simulink model "flexcan_can_fd_master_s32k14_Main_1"  (R2017a)
settings: Solver=FixedStepDiscrete  StartTime=0.0  StopTime=10.0  FixedStep=0.1  RelTol=1e-3  EnableMultiTasking=on
InitFcn:
  | mbd_s32k14_consistency_checks(bdroot(gcs));
undefined symbols (not defined in the file): A9, AD0, B8, C10, C2, C7, D1, D2, H6, PTA0, PTA2, PTC15, PTC6, PTC7, PTD0, PTE4, PTE5
libraries: mbd_s32k14_ec_toolbox x9
Description:
  | This model tests FlexCAN communication using CAN with Flexible Data-Rate.
  | The FlexCAN Master sends on each step a message with ID 0x3FF to the slave.
  | On each Tx Complete event Blue LED (PTD0) is toggled.
  | 
  | HW prerequisite:
  | - S32K144EVB-Q100
  | - Make sure that J107 has pin 1 and 2 connected and external power supply is provieded through J16.
  | 
  | Validation:
  | - The CAN Baudrate is set to 500 Kb/s
  | - Any CAN analizer (USB to CAN device) can be used to observe CAN traffic via board CAN port J13.
settings Model: Creator=agrigorev  LastModifiedBy=sreer
settings DataIOCC: ExternalInput=off  InitialState=off  LimitDataPoints=on  SaveFormat=Array  SaveOutput=off  SignalLogging=off  SaveTime=off
settings OptimizationCC: DefaultParameterBehavior=Inlined  PassReuseOutputArgsAs=Individual arguments
settings DebuggingCC: UnderspecifiedInitializationDetection=Classic  MergeDetectMultiDrivingBlocksExec=none  SolverPrmCheckMsg=warning  InheritedTsInSrcMsg=none  SingleTaskRateTransMsg=error  ParameterTunabilityLossMsg=error  UnconnectedInputMsg=error  UnconnectedOutputMsg=error  UnconnectedLineMsg=error  AllowSymbolicDim=off  UnknownTsInhSupMsg=error  StateNameClashWarn=warning  SFUnexpectedBacktrackingDiag=warning  SFNoUnconditionalDefaultTransitionDiag=warning  SFExecutionAtInitializationDiag=none
settings HardwareCC: ProdBitPerPointer=32  ProdBitPerSizeT=32  ProdBitPerPtrDiffT=32  ProdLargestAtomicInteger=Long  ProdLargestAtomicFloat=Double  ProdWordSize=32  ProdHWDeviceType=ARM Compatible->ARM Cortex
settings ModelReferenceCC: PropagateSignalLabelsOutOfModel=off
settings SFSimCC: MATLABDynamicMemAlloc=off
settings RTWCC: SystemTargetFile=mbd_s32k14.tlc  MakeCommand=mbd_s32k14_make_rtw COPY_MDLREF_INCLUDES=0  TemplateMakefile=mbd_s32k14.tmf  Description=Model Based Design Toolbox S32K14x Code Generation Target  GenerateReport=on  IncludeHyperlinkInReport=on  LaunchReport=on  GenerateTraceInfo=on  GenerateTraceReport=on  GenerateTraceReportSl=on  GenerateTraceReportSf=on  GenerateTraceReportEml=on
settings CodeAppCC: ForceParamTrailComments=on  IgnoreCustomStorageClasses=off  OperatorAnnotations=on  SimulinkDataObjDesc=on  SFDataObjDesc=on  MATLABFcnDesc=on  InsertBlockDesc=on  MATLABSourceComments=on
settings STFCustomTargetCC: MultiwordLength=256  CombineOutputUpdateFcns=on  ERTCustomFileBanners=on  SupportContinuousTime=off  SupportNonInlinedSFcns=off  RemoveResetFunc=on  MATLABClassNameForMDSCustomization=Simulink.SoftwareTarget.ERTCustomization  GRTInterface=off  SystemTargetFile=mbd_s32k14.tlc
settings ERTTargetCC: ParMdlRefBuildCompliant=off  CompOptLevelCompliant=off  ConcurrentExecutionCompliant=off  ERTFirstTimeCompliant=off  ModelStepFunctionPrototypeControlCompliant=off  CPPClassGenCompliant=off  UseToolchainInfoCompliant=off  InlinedParameterPlacement=NonHierarchical  ERTCustomFileTemplate=example_file_process.tlc
settings ConfigComp: CovMetricSettings=dw  CovHtmlReporting=on  CovSaveCumulativeToWorkspaceVar=on  CovSaveSingleToWorkspaceVar=on  CovExternalEMLEnable=off

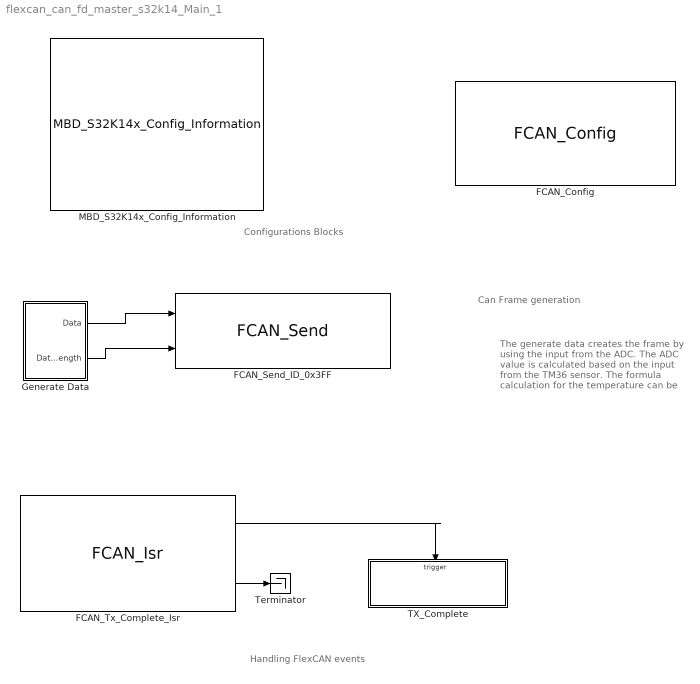
== system flexcan_can_fd_master_s32k14_Main_1 ==
  note: Handling FlexCAN events
  note: The generate data creates the frame by using the input from the ADC. The ADC value is calculated based on the input from the TM36 sensor. The formula calculation for the temperature can be
  note: Can Frame generation
  note: Configurations Blocks
  FCAN_Config : mbd_s32k14_ec_toolbox/S32K14x/Communication Blocks/Flex CAN Blocks/FCAN_Config  Priority=1  can_instance=0  can_mode=Normal mode  can_max_num_mb=16  can_rx=PTE4 : [9] : [6] : [D1]  can_tx=PTE5 : [8] : [5] : [D2]  show_adv_opts=on  can_clk_src=Peripheral clock  can_presdiv=9  can_rjw=0  can_pseg1=3  can_pseg2=3  can_propseg=6  can_cbt_presdiv=9  can_cbt_rjw=0  can_cbt_pseg1=3  can_cbt_pseg2=3  can_cbt_propseg=6  can_fd_enable=on  can_payload=8  can_rxfifo_enable=off  can_fifo_id_filter_extended=off  can_fifo_id_filter_remote=off  can_num_id_filters=8  can_fifo_id_format=A  can_fifo_id_filter={'0x0', '0x0', '0x0', '0x0', '0x0', '0x0', '0x0', '0x0'}  can_pn_enable=off  can_wakeup_match=off  can_wakeup_timeout=off  can_timeout_en=off  can_match_timeout=1  can_multiple_matches_en=off  can_num_matches=1  can_idfilter_extendedid=off  can_idfilter_remoteframe=off  can_idfilter_type=Match exact  can_idfilter_id1=0  can_idfilter_id2=0  can_payloadfilter_enable=off  can_payloadfilter_dlclow=0  can_payloadfilter_dlchigh=0  can_payloadfilter_type=Match exact  can_payloadfilter_payload1_b0=0  can_payloadfilter_payload1_b1=0  can_payloadfilter_payload1_b2=0  can_payloadfilter_payload1_b3=0  can_payloadfilter_payload1_b4=0  can_payloadfilter_payload1_b5=0  can_payloadfilter_payload1_b6=0  can_payloadfilter_payload1_b7=0  can_payloadfilter_payload2_b0=0  can_payloadfilter_payload2_b1=0  can_payloadfilter_payload2_b2=0  can_payloadfilter_payload2_b3=0  can_payloadfilter_payload2_b4=0  can_payloadfilter_payload2_b5=0  can_payloadfilter_payload2_b6=0  can_payloadfilter_payload2_b7=0
  FCAN_Send_ID_0x3FF : mbd_s32k14_ec_toolbox/S32K14x/Communication Blocks/Flex CAN Blocks/FCAN_Send  Priority=2  can_instance=0  can_mode=Non-blocking  can_timeout_ms=0  can_mb_idx=15  can_extended_id=off  can_is_remote=off  can_id=3FF  show_adv_opts=on  can_fd_enable=on  can_enable_brs=off  can_fd_padding=0
  FCAN_Tx_Complete_Isr : mbd_s32k14_ec_toolbox/S32K14x/Communication Blocks/Flex CAN Blocks/FCAN_Isr  can_instance=0  can_event=Tx Complete
  Generate Data : Subsystem
  MBD_S32K14x_Config_Information : mbd_s32k14_ec_toolbox/S32K14x/MBD_S32K14x_Config_Information  disp_str=|  config_params=[]
      | Target : S32K144-64KB_SRAM
      | Package : 100-pin
      | System clock : 80 MHz
      | XTAL clock : External 8 MHz
      | Compiler : GCC
      | Target Type : FLASH
      | Download Code after build : (OpenSDA: I)
      | Step Tick Interrupt Priority : 15
  TX_Complete : Subsystem  TreatAsAtomicUnit=on
      settings: RTWSystemCode=Nonreusable function
  Terminator : Terminator
  wires:
  FCAN_Tx_Complete_Isr/1 -> TX_Complete/Trigger
  FCAN_Tx_Complete_Isr/2 -> Terminator/1
  Generate Data/1(Data) -> FCAN_Send_ID_0x3FF/1
  Generate Data/2(Data Length) -> FCAN_Send_ID_0x3FF/2

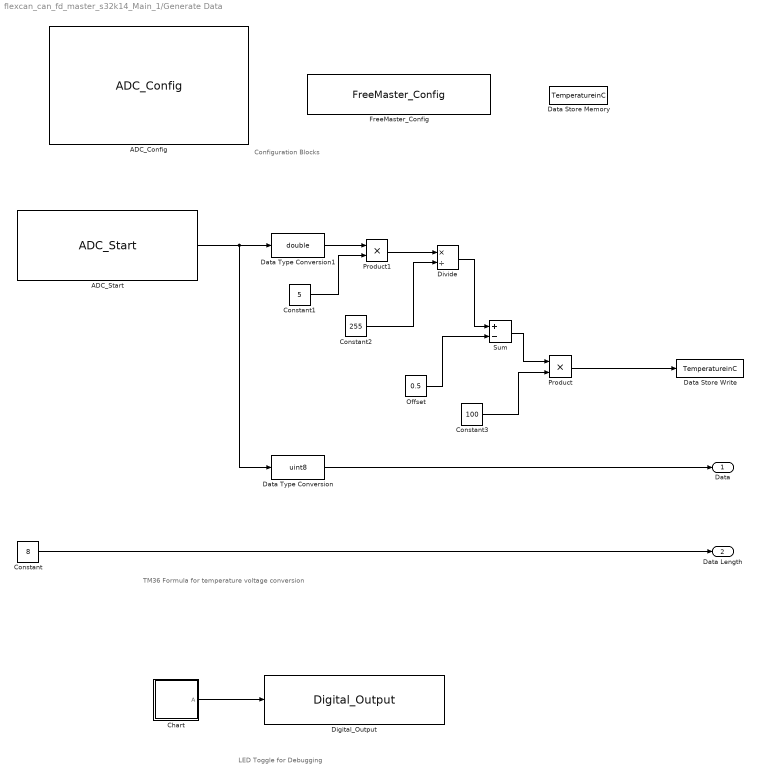
== system flexcan_can_fd_master_s32k14_Main_1/Generate Data ==
  note: LED Toggle for Debugging
  note: TM36 Formula for temperature voltage conversion
  note: Configuration Blocks
  ADC_Config : mbd_s32k14_ec_toolbox/S32K14x/Motor Control Blocks/ADC Blocks/ADC_Config  Priority=1  instance=0  mode=8-bit conversion  smplts=29  adiclk=alternate clock 1  adiv=input clock  show_adv_opts=on  pretrgsel=Software pre-trigger  swpretrg=Disabled  adtrg=software  trgsel=PDB output  refsel=Vrefh and Vrefl  acfe=off  acfgt=off  acren=off  cv1=0  cv2=0  adco=off  avge=off  avgs=4 samples
  ADC_Start : mbd_s32k14_ec_toolbox/S32K14x/Motor Control Blocks/ADC Blocks/ADC_Start  Priority=2  instance=0  adc_r=A  adc0_chan=PTA0 : [79] : [50] : [A9] : AD0  adc1_chan=PTA2 : [73] : [48] : [C10] : AD0  aien=off  mcuTargetUpdate=on
  Chart : Stateflow chart  TreatAsAtomicUnit=on
  Constant : Constant  Value=8  OutDataTypeStr=uint8
  Constant1 : Constant  Value=5  OutDataTypeStr=double
  Constant2 : Constant  Value=255  OutDataTypeStr=double
  Constant3 : Constant  Value=100  OutDataTypeStr=double
  Data Store Memory : DataStoreMemory  DataStoreName=TemperatureinC  ReadBeforeWriteMsg=warning  WriteAfterWriteMsg=warning  WriteAfterReadMsg=warning  ShowAdditionalParam=off  OutDataTypeStr=double
  Data Store Write : DataStoreWrite  DataStoreName=TemperatureinC
  Data Type Conversion : DataTypeConversion  OutDataTypeStr=uint8
  Data Type Conversion1 : DataTypeConversion  OutDataTypeStr=double
  Digital_Output : mbd_s32k14_ec_toolbox/S32K14x/Peripheral Interface Blocks/Digital_Output  gpio_pin=PTC15 : [45] : [29] : [H6]  port=C  pin=15  drive_strength=Low  slew_rate=Fast
  Divide : Product  Inputs=*/  OutDataTypeStr=double
  FreeMaster_Config : mbd_s32k14_ec_toolbox/S32K14x/Utility Blocks/FreeMaster_Config  interface=UART1  baudrate=115200  rxd=PTC6 : [81] : [52] : [C7]  txd=PTC7 : [80] : [51] : [B8]  mode=Short Interrupt  isr_prio=15  show_adv_opts=off  use_scope=on  max_scope_vars=8  use_recorder=on  max_rec_vars=8  rec_buff_size=1024  rec_timebase=0 milliseconds  comm_buffer_size_auto=on  comm_buffer_size=255  comm_rqueue_size_default=on  comm_rqueue_size=32
  Offset : Constant  Value=0.5  OutDataTypeStr=double
  Product : Product  OutDataTypeStr=double
  Product1 : Product  OutDataTypeStr=double  InputSameDT=on
  Sum : Sum  Inputs=+-  AccumDataTypeStr=double  OutDataTypeStr=double
  Data : Outport
  Data Length : Outport  Port=2
  wires:
  Constant/1 -> Data Length/1
  Chart/1(" A") -> Digital_Output/1
  ADC_Start/1 -> Data Type Conversion/1, Data Type Conversion1/1
  Data Type Conversion/1 -> Data/1
  Constant1/1 -> Product1/2
  Divide/1 -> Sum/1
  Offset/1 -> Sum/2
  Sum/1 -> Product/1
  Constant3/1 -> Product/2
  Product/1 -> Data Store Write/1
  Data Type Conversion1/1 -> Product1/1
  Product1/1 -> Divide/1
  Constant2/1 -> Divide/2

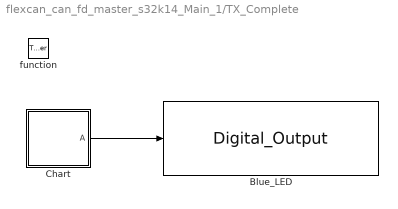
== system flexcan_can_fd_master_s32k14_Main_1/TX_Complete ==
  function : TriggerPort  TriggerType=function-call  VariantControl=Variant
  Blue_LED : mbd_s32k14_ec_toolbox/S32K14x/Peripheral Interface Blocks/Digital_Output  gpio_pin=PTD0 : [4] : [2] : [C2]  port=D  pin=0  drive_strength=Low  slew_rate=Fast
  Chart : Stateflow chart  TreatAsAtomicUnit=on
  wires:
  Chart/1(" A") -> Blue_LED/1

== stateflow chart flexcan_can_fd_master_s32k14_Main_1/Generate Data/Chart ==
  state A
  state A1
  (default) -> A
  A -> A1
  A1 -> A
  data: A output boolean [0..1]

== stateflow chart flexcan_can_fd_master_s32k14_Main_1/TX_Complete/Chart ==
  state A
  state A1
  (default) -> A
  A -> A1
  A1 -> A
  data: A output boolean [0..1]
